simulink model "EngDa_TEng"  (R2016b)
settings: configuration reference "CodeGenConfigSet" (kept outside this file)
undefined symbols (not defined in the file or in its folder): EngState_conv
settings Model: Creator=GaberXu  LastModifiedBy=lenovo
settings ConfigSetRef: SourceLocation=Base Workspace

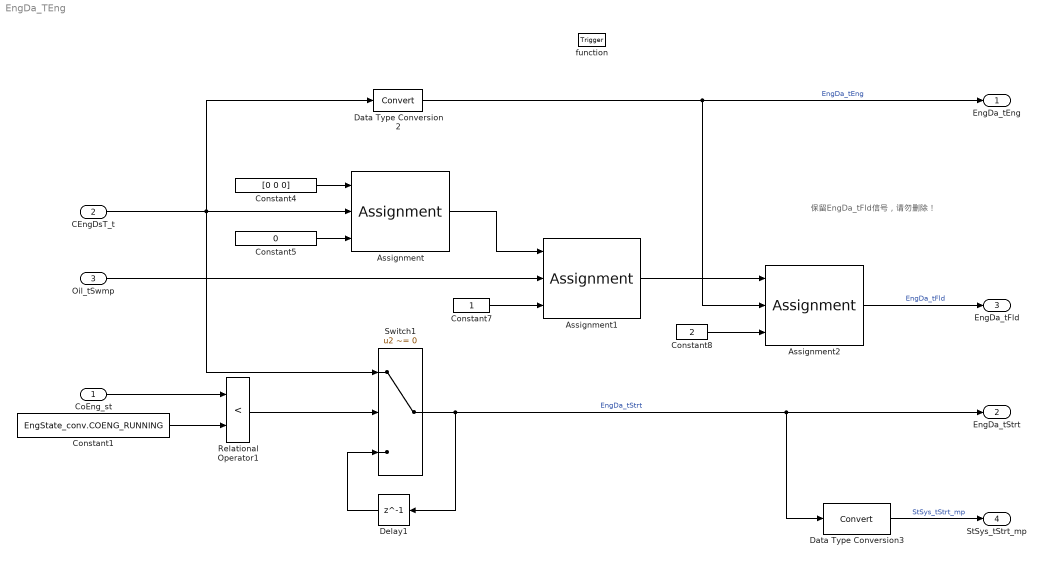
== system EngDa_TEng ==
  note: 保留EngDa_tFld信号，请勿删除！
  CoEng_st : Inport  Description=Engine coordinator state  OutDataTypeStr=Enum: EngState_conv
  CEngDsT_t : Inport  Tag=deg  Description=engine coolant temperature after filter  Port=2  OutMin=-200  OutMax=200  OutDataTypeStr=Temp_deg
  Oil_tSwmp : Inport  Tag=deg  Description=Oil temperature in oil sump  Port=3  OutMin=-50  OutMax=200  OutDataTypeStr=Temp_deg
  function : TriggerPort  TriggerType=function-call  VariantControl=Variant
  Assignment : Assignment  IndexMode=Zero-based  DiagnosticForDimensions=Warning  IndexOptions=Index vector (port)  Indices=1  OutputSizes=1
  Assignment1 : Assignment  IndexMode=Zero-based  DiagnosticForDimensions=Warning  IndexOptions=Index vector (port)  Indices=1  OutputSizes=1
  Assignment2 : Assignment  IndexMode=Zero-based  DiagnosticForDimensions=Warning  IndexOptions=Index vector (port)  Indices=1  OutputSizes=1
  Constant1 : Constant  Value=EngState_conv.COENG_RUNNING
  Constant4 : Constant  Value=[0 0 0]  OutDataTypeStr=Inherit: Inherit via back propagation
  Constant5 : Constant  Value=0  OutDataTypeStr=uint8
  Constant7 : Constant  OutDataTypeStr=uint8
  Constant8 : Constant  Value=2  OutDataTypeStr=uint8
  Data Type Conversion2 : DataTypeConversion
  Data Type Conversion3 : DataTypeConversion
  Delay1 : Delay  DelayLength=1  InitialCondition=0
  Relational Operator1 : RelationalOperator  Operator=<  OutDataTypeStr=boolean  RndMeth=Simplest
  Switch1 : Switch  Criteria=u2 ~= 0
  EngDa_tEng : Outport  Tag=deg  Description=Engine temperature  OutMin=-1000  OutMax=1000  OutDataTypeStr=Temp_deg
  EngDa_tStrt : Outport  Tag=deg  Description=Engine starting temperature  Port=2  OutMin=-1000  OutMax=1000  OutDataTypeStr=Temp_deg
  EngDa_tFld : Outport  Tag=deg  Description=Engine temperature field  Port=3  OutMin=-3000  OutMax=3000  OutDataTypeStr=Temp_deg
  StSys_tStrt_mp : Outport  Tag=deg  Description=engine temperature for starting system  Port=4  OutMin=-50  OutMax=150  OutDataTypeStr=Temp_deg
  wires:
  Assignment2/1 -> EngDa_tFld/1  "EngDa_tFld"
  Constant8/1 -> Assignment2/3
  Assignment1/1 -> Assignment2/1
  Constant7/1 -> Assignment1/3
  Assignment/1 -> Assignment1/1
  Constant5/1 -> Assignment/3
  Constant4/1 -> Assignment/1
  Delay1/1 -> Switch1/3
  Switch1/1 -> Data Type Conversion3/1, EngDa_tStrt/1, Delay1/1  "EngDa_tStrt"
  Relational Operator1/1 -> Switch1/2
  CoEng_st/1 -> Relational Operator1/1
  Constant1/1 -> Relational Operator1/2
  Data Type Conversion2/1 -> EngDa_tEng/1, Assignment2/2  "EngDa_tEng"
  Oil_tSwmp/1 -> Assignment1/2
  CEngDsT_t/1 -> Switch1/1, Assignment/2, Data Type Conversion2/1
  Data Type Conversion3/1 -> StSys_tStrt_mp/1  "StSys_tStrt_mp"
